simulink model "assignment_05"  (R2024a)
settings: Solver=VariableStepAuto  StartTime=0.0  StopTime=100.0  MaxStep=0.01  RelTol=1e-3
values from neighbouring files (symbols this model uses):
  B = input("enter the value of Dampaing factor: ")    [assignment_05_run.m]    (also in assignment_05_run_using_transfer_funcaiton.m)
  F = input("enter the value of Force: ")    [assignment_05_run.m]    (also in assignment_05_run_using_transfer_funcaiton.m)
  K = input("enter the value of K (Spring constant): ")    [assignment_05_run.m]    (also in assignment_05_run_using_transfer_funcaiton.m)
  M = input("enter the value of Mass: ")    [assignment_05_run.m]    (also in assignment_05_run_using_transfer_funcaiton.m)
settings Model: Creator=admin  LastModifiedBy=admin

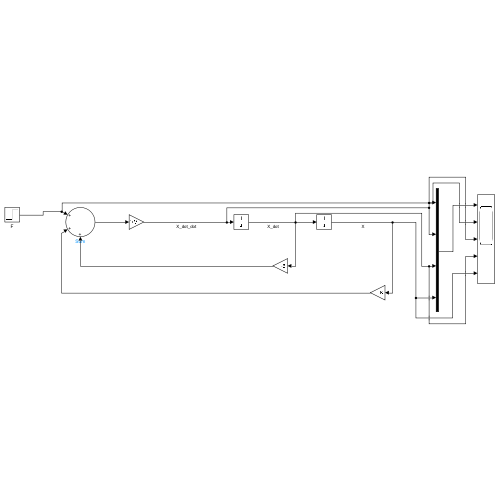
[thumbnail: Simulink's stored preview of the top-level diagram]
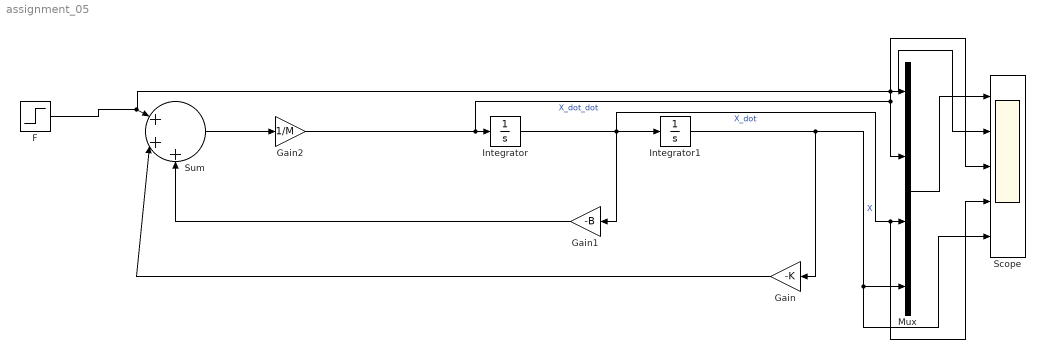
== system assignment_05 ==
  F : Step  After=F  SampleTime=0
  Gain : Gain  Gain=-K
  Gain1 : Gain  Gain=-B
  Gain2 : Gain  Gain=1/M
  Integrator : Integrator
  Integrator1 : Integrator
  Mux : Mux
  Scope : Scope  NumInputPorts=5
  Sum : Sum  Inputs=|+++
  wires:
  Gain2/1 -> Mux/2, Scope/3, Integrator/1  "X_dot_dot"
  Integrator/1 -> Gain1/1, Scope/4, Mux/3, Integrator1/1  "X_dot"
  Integrator1/1 -> Gain/1, Scope/5, Mux/4  "X"
  Sum/1 -> Gain2/1
  F/1 -> Scope/2, Mux/1, Sum/1
  Gain1/1 -> Sum/3
  Gain/1 -> Sum/2
  Mux/1 -> Scope/1
